simulink model "VB_RIFKF_GNSS_INS25"  (R2023a)
settings: Solver=FixedStepAuto  StartTime=0  StopTime=500  FixedStep=0.01  RelTol=1e-3
InitFcn:
  | resilient_initNavigation1216;
  | init_param;
undefined symbols (not defined in the file or in its folder): dt, g0, gam0_rad, ISUS_flag, magnitude, p, P0, P0_RIEKF, param, pd0, pe0, phi0_rad, pn0, psi, psi0_rad, state_dim, vd0, ve0, vn0
libraries: simulink_extras x68, dspstat3 x54, sharedtransform x47, simulink x43, matrix_library x9, sharedTrackingLibrary x5, dspfactors x4, aerolibconvert2 x3, aerolibtransform2 x3
(part 18 of 22)

== matlab function VB_RIFKF_GNSS_INS25/ER EKF/INS propogation/Init_PVQ/Horizontal_attitude2/Hem2JPL2 ==
  data: q input; y output
function y = fcn(q)

y = [q(2:4);q(1)];

== matlab function VB_RIFKF_GNSS_INS25/ER EKF/INS propogation/att_update/JPLQuatMult ==
  data: quatA input; q_t output; quatB input
function q_t = QuatMult(quatA,quatB)
% Calculate the following quaternion product quatA * quatB using the 
% standard identity 
%{
inline Eigen::Matrix<double, 4, 1> quat_multiply(const Eigen::Matrix<double, 4, 1> &q, const Eigen::Matrix<double, 4, 1> &p) {
  Eigen::Matrix<double, 4, 1> q_t;
  Eigen::Matrix<double, 4, 4> Qm;
  // create big L matrix
  Qm.block(0, 0, 3, 3) = q(3, 0) * Eigen::MatrixXd::Identity(3, 3) - skew_x(q.block(0, 0, 3, 1));
  Qm.block(0, 3, 3, 1) = q.block(0, 0, 3, 1);
  Qm.block(3, 0, 1, 3) = -q.block(0, 0, 3, 1).transpose();
  Qm(3, 3) = q(3, 0);
  q_t = Qm * p;
  // ensure unique by forcing q_4 to be >0
  if (q_t(3, 0) < 0) {
    q_t *= -1;
  }
  // normalize and return
  return q_t / q_t.norm();
}
%}
Qm = zeros(4,4);
q_t = zeros(4,1);
Qm(1:3,1:3) = quatA(4)*eye(3,3) - skewMat(quatA(1:3));
Qm(1:3,4) = quatA(1:3);
Qm(4,1:3) = -quatA(1:3)';
Qm(4,4) = quatA(4);
q_t = Qm * quatB;
if q_t(4) < 0
    q_t = q_t * (-1);
end
q_t = q_t / norm(q_t);
end

== matlab function VB_RIFKF_GNSS_INS25/ISUS_RIEKF3/INS propogation3/vel//pos update/pos update/MATLAB Function ==
  data: dtheta input; pos_correct output single; KFState_dp input; pos input
function pos_correct = fcn(dtheta, KFState_dp, pos)
    
     pos_correct =  KFState_dp + exp_so3(dtheta)*pos;
    %pos_correct = pos + KFState_dp - skewMat(pos)*dtheta;
    
end

== matlab function VB_RIFKF_GNSS_INS25/ER EKF/INS propogation/att_update/JPLQuatMult1 ==
  data: quatA input; q_t output; quatB input
function q_t = QuatMult(quatA,quatB)
% Calculate the following quaternion product quatA * quatB using the 
% standard identity 
%{
inline Eigen::Matrix<double, 4, 1> quat_multiply(const Eigen::Matrix<double, 4, 1> &q, const Eigen::Matrix<double, 4, 1> &p) {
  Eigen::Matrix<double, 4, 1> q_t;
  Eigen::Matrix<double, 4, 4> Qm;
  // create big L matrix
  Qm.block(0, 0, 3, 3) = q(3, 0) * Eigen::MatrixXd::Identity(3, 3) - skew_x(q.block(0, 0, 3, 1));
  Qm.block(0, 3, 3, 1) = q.block(0, 0, 3, 1);
  Qm.block(3, 0, 1, 3) = -q.block(0, 0, 3, 1).transpose();
  Qm(3, 3) = q(3, 0);
  q_t = Qm * p;
  // ensure unique by forcing q_4 to be >0
  if (q_t(3, 0) < 0) {
    q_t *= -1;
  }
  // normalize and return
  return q_t / q_t.norm();
}
%}
Qm = zeros(4,4);
q_t = zeros(4,1);
Qm(1:3,1:3) = quatA(4)*eye(3,3) - skewMat(quatA(1:3));
Qm(1:3,4) = quatA(1:3);
Qm(4,1:3) = -quatA(1:3)';
Qm(4,4) = quatA(4);
q_t = Qm * quatB;
if q_t(4) < 0
    q_t = q_t * (-1);
end
q_t = q_t / norm(q_t);
end

== matlab function VB_RIFKF_GNSS_INS25/ER EKF/INS propogation/att_update/JPLrv2q ==
  data: rotVec input; quaternion output
% convert froma rotation vector in radians to a quaternion
function quaternion = RotToQuat(rotVec)

vecLength = sqrt(rotVec(1)^2 + rotVec(2)^2 + rotVec(3)^2);

if vecLength < 1e-6
  quaternion = [0;0;0;1];
else
  quaternion = [rotVec/vecLength*sin(0.5*vecLength);cos(0.5*vecLength);];
end

== matlab function VB_RIFKF_GNSS_INS25/ER EKF/INS propogation/att_update/JPLrv2q1 ==
  data: deltaTheta input; updateQuat output
% convert froma rotation vector in radians to a quaternion
function updateQuat = RotToQuat(deltaTheta)

    deltaq = 0.5 * deltaTheta;
    
    checkNorm = deltaq' * deltaq;
    
    if checkNorm > 1
        updateQuat = [deltaq; 1];
        updateQuat = updateQuat / sqrt(1 + checkNorm);
    else
        updateQuat = [deltaq; sqrt(1 - checkNorm)];
    end
    
    updateQuat = updateQuat / norm(updateQuat);
end

== matlab function VB_RIFKF_GNSS_INS25/ER EKF/INS propogation/att_update/MATLAB Function1 ==
  data: q input; Rot output
function Rot = quat_2_Rot(q)

%{
inline Eigen::Matrix<double, 3, 3> quat_2_Rot(const Eigen::Matrix<double, 4, 1> &q) {
  Eigen::Matrix<double, 3, 3> q_x = skew_x(q.block(0, 0, 3, 1));
  Eigen::MatrixXd Rot = (2 * std::pow(q(3, 0), 2) - 1) * Eigen::MatrixXd::Identity(3, 3) - 2 * q(3, 0) * q_x +
                        2 * q.block(0, 0, 3, 1) * (q.block(0, 0, 3, 1).transpose());
  return Rot;
}
%}
q_x = skewMat(q(1:3));
Rot = (2 * q(4)^2 - 1) * eye(3, 3) - 2 * q(4) * q_x +...
       2 * q(1:3) * q(1:3)';
end

== matlab function VB_RIFKF_GNSS_INS25/ISUS_RIEKF3/Error State Kalman Filter M1/Extended Kalman Filter M1/Correct M1/Correct ==
  settings: updateMethod=DISCRETE  sampleTime=SampleTime
  data: x input; xNew output; P input; P output; yMeas input; R input; uMeas input; blockOrdering input; pM parameter; blockOrdering output
function [xNew,P,blockOrdering] = fcn(x,P,yMeas,R,uMeas,blockOrdering,pM)
% ekfCorrect Correction step for EKF
%
%   Copyright 2016-2021 The MathWorks, Inc.

%#codegen

% If measurement noise is time-varying then compute square-root
% factorization.
if pM.HasTimeVaryingR
   R = matlabshared.tracking.internal.svdPSD(R);
end

% Construct the function handle for measurement fcn
if pM.IsSimulinkFcn
    MeasurementFcnH_SL = str2func(pM.FcnName);
    if pM.HasAdditiveNoise
        MeasurementFcnH = @(fState)MeasurementFcnH_SL(fState);
    else
        MeasurementFcnH = @(fState,fMeasNoise)MeasurementFcnH_SL(fState,fMeasNoise);
    end
else
    MeasurementFcnH = str2func(pM.FcnName);
end

% Construct the function handle for measurement Jacobian fcn
if pM.HasJacobian
    if pM.IsSimulinkFcn
        MeasurementJacobianFcnH_SL = str2func(pM.JacobianFcnName);
        if pM.HasAdditiveNoise
            MeasurementJacobianFcnH = @(fState)MeasurementJacobianFcnH_SL(fState);
        else
            MeasurementJacobianFcnH = @(fState,fMeasNoise)MeasurementJacobianFcnH_SL(fState,fMeasNoise);
        end
    else
        MeasurementJacobianFcnH = str2func(pM.JacobianFcnName);
    end
else
    MeasurementJacobianFcnH = [];
end

% Handle (optional) extra input arguments of the measurement & jacobian fcns
switch pM.NumberOfExtraArgumentInports
    case 0
        extraArgs = {};
    case 1
        extraArgs = {uMeas};
    otherwise
        assert(false);
end

% Construct the corrector, perform the update
if pM.HasAdditiveNoise
    ekfCorrector = matlabshared.tracking.internal.EKFCorrectorAdditive();
else
    ekfCorrector = matlabshared.tracking.internal.EKFCorrectorNonAdditive();
end

% Check if dimensions and type of Measurement and Jacobian are correct
if pM.HasAdditiveNoise
   % Additive noise
   
   % MeasurementFcn
   ztry = MeasurementFcnH(x, extraArgs{:});
   
   if pM.IsSimulinkFcn
      hasError = (numel(ztry) ~= numel(yMeas));
   else
      hasError = (numel(ztry) ~= numel(yMeas)) || ~isa(ztry, class(x));
   end
   
   coder.internal.errorIf(...
      hasError,...
      'shared_tracking:ExtendedKalmanFilter:MeasurementNonMatchingSizeOrClass',...
      'MeasurementFcn');
   
   if pM.HasJacobian
      % MeasurementJacobianFcn
      Htry = MeasurementJacobianFcnH(x, extraArgs{:});
      isSizeNotCorrect = numel(yMeas) ~= size(Htry,1) || numel(x) ~= size(Htry,2);
      
      if pM.IsSimulinkFcn
         hasError = isSizeNotCorrect;
      else
         hasError = isSizeNotCorrect || ~isa(Htry, class(x));
      end
      
      coder.internal.errorIf(...
         hasError,...
         'shared_tracking:ExtendedKalmanFilter:MeasurementJacobianNonMatchingSizeOrClass',...
         'MeasurementJacobianFcn',numel(yMeas),numel(x));
   end   
else
   % Non-additive noise
   
   % MeasurementFcn
   ztry = MeasurementFcnH(...
      x, zeros(size(R,1),1,'like',x), ...
      extraArgs{:});   

   if pM.IsSimulinkFcn
      hasError = (numel(ztry) ~= numel(yMeas));
   else
      hasError = (numel(ztry) ~= numel(yMeas)) || ~isa(ztry, class(x));
   end
   
   coder.internal.errorIf(...
      hasError,...
      'shared_tracking:ExtendedKalmanFilter:MeasurementNonMatchingSizeOrClass',...
      'MeasurementFcn');
   
   if pM.HasJacobian
      % MeasurementJacobianFcn
      Htry = MeasurementJacobianFcnH(...
         x, zeros(size(R,1),1,'like',x), ...
         extraArgs{:});
      
      isSizeNotCorrect = numel(yMeas) ~= size(Htry,1) || numel(x) ~= size(Htry,2);     
      
      if pM.IsSimulinkFcn
         hasError = isSizeNotCorrect;
      else
         hasError = isSizeNotCorrect || ~isa(Htry, class(x));
      end
      
      coder.internal.errorIf(...
         hasError,...
         'shared_tracking:ExtendedKalmanFilter:MeasurementJacobianNonMatchingSizeOrClass',...
         'MeasurementJacobianFcn',numel(yMeas),numel(x));
   end
end
% Measurement wrapping
ekfCorrector.HasMeasurementWrapping = pM.HasWrapping;

xNew = zeros(size(x),'like',x); %#ok<PREALL>
% wk = 0;
[xNew,P] = ekfCorrector.correct(...
        yMeas,R,x,P,MeasurementFcnH,MeasurementJacobianFcnH,extraArgs{:});
end

== matlab function VB_RIFKF_GNSS_INS25/ISUS_RIEKF3/Error State Kalman Filter M1/Extended Kalman Filter M1/Correct M1/MATLAB Function ==
  data: u input; y output
function y = fcn(u)

y = tril(u);

== matlab function VB_RIFKF_GNSS_INS25/ISUS_RIEKF3/Error State Kalman Filter M1/Extended Kalman Filter M1/Correct M1/Subsystem2/MATLAB Function1 ==
  data: u input; y output; X input; ISUS_flag input
function y = fcn(u, X, ISUS_flag)
if ISUS_flag == 0
    y = X;
else
     y = u;
    %y(1:9,1:9) = u;
end

== matlab function VB_RIFKF_GNSS_INS25/ISUS_RIEKF3/Error State Kalman Filter M1/Extended Kalman Filter M1/Correct M1/innovation calculation/MATLAB Function ==
  data: u input; y output
function y = fcn(u)

y = u*u';

== matlab function VB_RIFKF_GNSS_INS25/ISUS_RIEKF3/Error State Kalman Filter M1/Extended Kalman Filter M1/Output/MATLAB Function ==
  data: S input; P output
function P = fcn(S)
    
    % Get back Covariance from Square-root Covariance
    P = S*S';
    %P = 1/2*(S+S');
    
end

== matlab function VB_RIFKF_GNSS_INS25/ISUS_RIEKF3/Error State Kalman Filter M1/Extended Kalman Filter M1/Predict/Predict ==
  settings: updateMethod=DISCRETE  sampleTime=SampleTime
  data: x input; xNew output; P input; Q input; uState input; unused input; P output; pS parameter
function [xNew,P] = fcn(x,P,Q,uState,~,pS)
% ekfCorrect Prediction step for EKF
%
%   Copyright 2016-2021 The MathWorks, Inc.

%#codegen

% If process noise is time-varying then compute square-root
% factorization.
if pS.HasTimeVaryingQ
   Q = matlabshared.tracking.internal.svdPSD(Q);
end

% Construct fcn handles
if pS.IsSimulinkFcn
    StateTransitionJacobianFcnH_SL = str2func(pS.FcnName);
    if pS.HasAdditiveNoise
        StateTransitionFcnH = @(fState)StateTransitionJacobianFcnH_SL(fState);
    else
        StateTransitionFcnH = @(fState,fProcNoise)StateTransitionJacobianFcnH_SL(fState,fProcNoise);
    end
else
    StateTransitionFcnH = str2func(pS.FcnName);
end
if pS.HasJacobian
    if pS.IsSimulinkFcn
        StateTransitionJacobianFcnH_SL = str2func(pS.JacobianFcnName);
        if pS.HasAdditiveNoise
            StateTransitionJacobianFcnH = @(fState)StateTransitionJacobianFcnH_SL(fState);
        else
            StateTransitionJacobianFcnH = @(fState,fProcNoise)StateTransitionJacobianFcnH_SL(fState,fProcNoise);
        end
    else
        StateTransitionJacobianFcnH = str2func(pS.JacobianFcnName);
    end
else
    StateTransitionJacobianFcnH = [];
end

switch pS.NumberOfExtraArgumentInports
    case 0
        extraArgs = {};
    case 1
        extraArgs = {uState};
    otherwise
        assert(false);
end

% Check if dimensions and type of State and Jacobian are correct
if pS.HasAdditiveNoise
   % Additive noise
   
   % StateTransitionFcn
   xTry = StateTransitionFcnH(x, extraArgs{:});
   
   if pS.IsSimulinkFcn
      hasError = any(size(x) ~= size(xTry));
   else
      hasError = any(size(x) ~= size(xTry)) || ~isa(xTry, class(x));
   end
   
   coder.internal.errorIf(...
      hasError,...
      'shared_tracking:ExtendedKalmanFilter:StateNonMatchingSizeOrClass',...
      'StateTransitionFcn', 'State', numel(x));
   
   if pS.HasJacobian
      % Jacobian
      F = StateTransitionJacobianFcnH(x, extraArgs{:});
      % F needs to be square
      isSizeNotCorrect = ~all(size(F) == numel(x));
      
      if pS.IsSimulinkFcn
         hasError = isSizeNotCorrect;
      else
         hasError = isSizeNotCorrect || ~isa(F, class(x));
      end
      
      coder.internal.errorIf(...
         hasError,...
         'shared_tracking:ExtendedKalmanFilter:StateTransitionJacobianNonMatchingSizeOrClass',...
         'StateTransitionJacobianFcn', numel(x));
   end
else
   % Non-additive noise
   
   % StateTransitionFcn
   xTry = StateTransitionFcnH(x, zeros(size(Q,1),1,'like',x),extraArgs{:});
   
   if pS.IsSimulinkFcn
      hasError = any(size(x) ~= size(xTry));
   else
      hasError = any(size(x) ~= size(xTry)) || ~isa(xTry, class(x));
   end
   
   coder.internal.errorIf(...
      hasError,...
      'shared_tracking:ExtendedKalmanFilter:StateNonMatchingSizeOrClass',...
      'StateTransitionFcn', 'State', numel(x))
   
   if pS.HasJacobian
      % Jacobian
      F = StateTransitionJacobianFcnH(x, zeros(size(Q,1),1,'like',x),extraArgs{:});
      % F needs to be square
      isSizeNotCorrect = ~all(size(F) == numel(x));
      
      if pS.IsSimulinkFcn
         hasError = isSizeNotCorrect;
      else
         hasError = isSizeNotCorrect || ~isa(F, class(x));
      end
       
      coder.internal.errorIf(...
         hasError,...
         'shared_tracking:ExtendedKalmanFilter:StateTransitionJacobianNonMatchingSizeOrClass',...
         'StateTransitionJacobianFcn', numel(x));
   end
end

xNew = zeros(size(x),'like',x); %#ok<PREALL>

if pS.HasAdditiveNoise
    [xNew,P] = matlabshared.tracking.internal.EKFPredictorAdditive.predict(...
        Q,x,P,StateTransitionFcnH,StateTransitionJacobianFcnH,extraArgs{:});
else    
    [xNew,P] = matlabshared.tracking.internal.EKFPredictorNonAdditive.predict(...
        Q,x,P,StateTransitionFcnH,StateTransitionJacobianFcnH,extraArgs{:});
end
end

== matlab function VB_RIFKF_GNSS_INS25/ISUS_RIEKF3/Error State Kalman Filter M1/Extended Kalman Filter M1/innovation calculation/MATLAB Function ==
  data: u input; y output
function y = fcn(u)

y = u*u';

== matlab function VB_RIFKF_GNSS_INS25/ER EKF/Error State Kalman Filter/Extended Kalman Filter2/Correct1/Correct ==
  settings: updateMethod=DISCRETE  sampleTime=SampleTime
  data: x input; xNew output; P input; P output; yMeas input; R input; uMeas input; blockOrdering input; pM parameter; blockOrdering output
function [xNew,P,blockOrdering] = fcn(x,P,yMeas,R,uMeas,blockOrdering,pM)
% ekfCorrect Correction step for EKF
%
%   Copyright 2016-2021 The MathWorks, Inc.

%#codegen

% If measurement noise is time-varying then compute square-root
% factorization.
if pM.HasTimeVaryingR
   R = matlabshared.tracking.internal.svdPSD(R);
end

% Construct the function handle for measurement fcn
if pM.IsSimulinkFcn
    MeasurementFcnH_SL = str2func(pM.FcnName);
    if pM.HasAdditiveNoise
        MeasurementFcnH = @(fState)MeasurementFcnH_SL(fState);
    else
        MeasurementFcnH = @(fState,fMeasNoise)MeasurementFcnH_SL(fState,fMeasNoise);
    end
else
    MeasurementFcnH = str2func(pM.FcnName);
end

% Construct the function handle for measurement Jacobian fcn
if pM.HasJacobian
    if pM.IsSimulinkFcn
        MeasurementJacobianFcnH_SL = str2func(pM.JacobianFcnName);
        if pM.HasAdditiveNoise
            MeasurementJacobianFcnH = @(fState)MeasurementJacobianFcnH_SL(fState);
        else
            MeasurementJacobianFcnH = @(fState,fMeasNoise)MeasurementJacobianFcnH_SL(fState,fMeasNoise);
        end
    else
        MeasurementJacobianFcnH = str2func(pM.JacobianFcnName);
    end
else
    MeasurementJacobianFcnH = [];
end

% Handle (optional) extra input arguments of the measurement & jacobian fcns
switch pM.NumberOfExtraArgumentInports
    case 0
        extraArgs = {};
    case 1
        extraArgs = {uMeas};
    otherwise
        assert(false);
end

% Construct the corrector, perform the update
if pM.HasAdditiveNoise
    ekfCorrector = matlabshared.tracking.internal.EKFCorrectorAdditive();
else
    ekfCorrector = matlabshared.tracking.internal.EKFCorrectorNonAdditive();
end

% Check if dimensions and type of Measurement and Jacobian are correct
if pM.HasAdditiveNoise
   % Additive noise
   
   % MeasurementFcn
   ztry = MeasurementFcnH(x, extraArgs{:});
   
   if pM.IsSimulinkFcn
      hasError = (numel(ztry) ~= numel(yMeas));
   else
      hasError = (numel(ztry) ~= numel(yMeas)) || ~isa(ztry, class(x));
   end
   
   coder.internal.errorIf(...
      hasError,...
      'shared_tracking:ExtendedKalmanFilter:MeasurementNonMatchingSizeOrClass',...
      'MeasurementFcn');
   
   if pM.HasJacobian
      % MeasurementJacobianFcn
      Htry = MeasurementJacobianFcnH(x, extraArgs{:});
      isSizeNotCorrect = numel(yMeas) ~= size(Htry,1) || numel(x) ~= size(Htry,2);
      
      if pM.IsSimulinkFcn
         hasError = isSizeNotCorrect;
      else
         hasError = isSizeNotCorrect || ~isa(Htry, class(x));
      end
      
      coder.internal.errorIf(...
         hasError,...
         'shared_tracking:ExtendedKalmanFilter:MeasurementJacobianNonMatchingSizeOrClass',...
         'MeasurementJacobianFcn',numel(yMeas),numel(x));
   end   
else
   % Non-additive noise
   
   % MeasurementFcn
   ztry = MeasurementFcnH(...
      x, zeros(size(R,1),1,'like',x), ...
      extraArgs{:});   

   if pM.IsSimulinkFcn
      hasError = (numel(ztry) ~= numel(yMeas));
   else
      hasError = (numel(ztry) ~= numel(yMeas)) || ~isa(ztry, class(x));
   end
   
   coder.internal.errorIf(...
      hasError,...
      'shared_tracking:ExtendedKalmanFilter:MeasurementNonMatchingSizeOrClass',...
      'MeasurementFcn');
   
   if pM.HasJacobian
      % MeasurementJacobianFcn
      Htry = MeasurementJacobianFcnH(...
         x, zeros(size(R,1),1,'like',x), ...
         extraArgs{:});
      
      isSizeNotCorrect = numel(yMeas) ~= size(Htry,1) || numel(x) ~= size(Htry,2);     
      
      if pM.IsSimulinkFcn
         hasError = isSizeNotCorrect;
      else
         hasError = isSizeNotCorrect || ~isa(Htry, class(x));
      end
      
      coder.internal.errorIf(...
         hasError,...
         'shared_tracking:ExtendedKalmanFilter:MeasurementJacobianNonMatchingSizeOrClass',...
         'MeasurementJacobianFcn',numel(yMeas),numel(x));
   end
end
% Measurement wrapping
ekfCorrector.HasMeasurementWrapping = pM.HasWrapping;

xNew = zeros(size(x),'like',x); %#ok<PREALL>
% wk = 0;
[xNew,P] = ekfCorrector.correct(...
        yMeas,R,x,P,MeasurementFcnH,MeasurementJacobianFcnH,extraArgs{:});
end

== matlab function VB_RIFKF_GNSS_INS25/ISUS_RIEKF3/Error State Kalman Filter M1/MATLAB Function ==
  data: u input; dp output size=3; dv output size=3; dtheta output size=3; da output size=3; dg output size=3
function [dp,dv,dtheta,da,dg] = fcn(u)
    dtheta = u(1:3);
    dv = u(4:6);
    dp = u(7:9);
    dg = u(10:12);
    da = u(13:15);

end

== matlab function VB_RIFKF_GNSS_INS25/ISUS_RIEKF1/INS propogation/att update/MATLAB Function ==
  data: Rbn_k_1 input; Rbn output; w input; dt input
function Rbn = fcn(Rbn_k_1, w, dt)
    Rbn =  Rbn_k_1 * exp_so3( w * dt);
end

== matlab function VB_RIFKF_GNSS_INS25/ISUS_RIEKF1/INS propogation/att update/MATLAB Function2 ==
  data: delta input; Rbn_correct output single size=[3,3]; Rbn input
function Rbn_correct = fcn(delta, Rbn)
    Rbn_correct = zeros(3,3);
     Rbn_correct = exp_so3(delta)* Rbn;
    %Rbn_correct =( eye(3) + skewMat(delta))* Rbn;
end

== matlab function VB_RIFKF_GNSS_INS25/ISUS_RIEKF1/INS propogation/vel//pos update/pos update/MATLAB Function ==
  data: dtheta input; pos_correct output single; KFState_dp input; pos input
function pos_correct = fcn(dtheta, KFState_dp, pos)
    
     pos_correct =  KFState_dp + exp_so3(dtheta)*pos;
    %pos_correct = pos + KFState_dp - skewMat(pos)*dtheta;
    
end

== matlab function VB_RIFKF_GNSS_INS25/ISUS_RIEKF1/INS propogation/vel//pos update/vel update/MATLAB Function ==
  data: dtheta input; vel_correct output single; KFState_dv input; vel input
function vel_correct = fcn(dtheta, KFState_dv, vel)
    
     vel_correct =  KFState_dv + exp_so3( dtheta)*vel;
    %vel_correct =  vel + KFState_dv - skewMat(vel)*dtheta;
end

== matlab function VB_RIFKF_GNSS_INS25/ISUS_RIEKF3/Error State Kalman Filter M1/Simulink Function - GPS Measurements/MATLAB Function ==
  data: vn input; H output; pn input
function H = fcn(vn, pn)
    state_dim = 15;
    H = zeros(6,state_dim);
    H(1:3,1:3) = skewMat(vn);
    H(4:6,1:3) = skewMat(pn);
    H(1:6,4:9) = eye(6);
    %H = -H;
end

== matlab function VB_RIFKF_GNSS_INS25/ISUS_RIEKF3/Error State Kalman Filter M1/Simulink Function - GPS Measurements/MATLAB Function1 ==
  data: Rbn input; vn input; X_inv output; pn input
function X_inv = invX(Rbn, vn, pn)
    X_inv = zeros(5,5);
    Rnb = Rbn';
    X_inv(1:3,1:3) = Rnb;
    X_inv(1:3,4) = -Rnb * vn;
    X_inv(1:3,5) = -Rnb * pn;
    X_inv(4:5,4:5) = eye(2);
end

== matlab function VB_RIFKF_GNSS_INS25/ISUS_RIEKF3/Error State Kalman Filter M1/Simulink Function - GPS Measurements1/MATLAB Function ==
  data: vn input; H_baro output; pn input
function H_baro = fcn(vn, pn)
    state_dim = 24;
    H = zeros(6,state_dim);
    H(1:3,1:3) = skewMat(vn);
    H(4:6,1:3) = skewMat(pn);
    H(1:6,4:9) = eye(6);
    
    A = [0 0 0 0 0 1];
    H_baro = A * H;
end

== matlab function VB_RIFKF_GNSS_INS25/ISUS_RIEKF3/Error State Kalman Filter M1/Simulink Function - GPS Measurements2/MATLAB Function ==
  data: Rbn input; Magn input; H output; dtheta input
function H = fcn(Rbn, Magn, dtheta)
    state_dim = 24;
    H = zeros(3,state_dim);
    H(1:3,1:3) =  Rbn * skewMat(Magn);
    H(1:3,16:18) =  Rbn * skewMat(dtheta);
end

== matlab function VB_RIFKF_GNSS_INS25/ISUS_RIEKF3/Error State Kalman Filter M1/Simulink Function - GPS Measurements3/MATLAB Function ==
  data: Rbn input; Rab input; H output; vn input; v_wind input
function H = fcn(Rbn,Rab, vn,v_wind)
    state_dim = 24;
    A = Rab' * Rbn';
    H = zeros(3,state_dim);
   % H(1:3,1:3) =  - skewMat(vn - v_wind);
   % H(1:3,4:6) =  eye(3);
    H(1:3,19:21) =  - skewMat(vn - v_wind);
    H(1:3,22:24) =  - eye(3);
    H = double(A * H);
end

== matlab function VB_RIFKF_GNSS_INS25/ISUS_RIEKF3/Error State Kalman Filter M1/Simulink Function - State Transition/Cal Phi/MATLAB Function1 ==
  data: vn input; Phi output; pn input; Rbn input; dt input
function Phi = fcn(vn,pn, Rbn,dt)
    state_dim = 15;
    %{
    F.block(0, 0, 3, 3) = exp_so3(-w_hat * dt);
        F.block(0, 9, 3, 3).noalias() = -exp_so3(-w_hat * dt) * Jr_so3(-w_hat * dt) * dt;
        F.block(9, 9, 3, 3).setIdentity();
        F.block(6, 0, 3, 3).noalias() = -R_Gtoi.transpose() * skew_x(a_hat * dt);
        F.block(6, 6, 3, 3).setIdentity();
        F.block(6, 12, 3, 3) = -R_Gtoi.transpose() * dt;
        F.block(12, 12, 3, 3).setIdentity();
        F.block(3, 0, 3, 3).noalias() = -0.5 * R_Gtoi.transpose() * skew_x(a_hat * dt * dt);
        F.block(3, 6, 3, 3) = Eigen::Matrix3d::Identity() * dt;
        F.block(3, 12, 3, 3) = -0.5 * R_Gtoi.transpose() * dt * dt;
        F.block(3, 3, 3, 3).setIdentity();
        Eigen::Matrix<double, 15, 12> G = Eigen::Matrix<double, 15, 12>::Zero();
    %}
    %
    %
    %F = [0_33         0_33  0_33   -Rbn          0_33]
    %    [skew(gn)     0_33  0_33  -skew(vn)Rbn   -Rbn]
    %    [0.5*skew(gn) I_33  0_33  -skew(pn)Rbn   -Rbn]
    %    [         0_69                  I66          ]
    %
    %0611 yxy
        %F = [0_33         0_33  0_33   -Rbn          0_33]
    %    [skew(gn)     0_33  0_33  -skew(vn)Rbn   Rbn]
    %    [0.5*skew(gn) I_33  0_33  -skew(pn)Rbn   Rbn]
    %    [         0_69                  I66          ]
    Phi = zeros(state_dim,state_dim);
    g0 = 9.79;
    gn = [0;0;-g0];
    tao_wind = 50;
    F  = zeros(state_dim,state_dim);
    F(1:3,10:12) = -Rbn;
    F(4:6,1:3)   = skewMat(gn);
    F(4:6,10:12) = -skewMat(vn)*Rbn;
    F(4:6,13:15) = -Rbn*(-1);
    F(7:9,4:6)   = eye(3);
    F(7:9,1:3)   = 0.5*skewMat(gn)*dt;
    F(7:9,10:12) = -skewMat(pn)*Rbn;
    F(7:9,13:15) = -Rbn*(-1);
    %F(10:15,10:15) = eye(6);
    % F(22:24,22:24) = -1/tao_wind;
    Phi = eye(state_dim) + F * dt;

end

== matlab function VB_RIFKF_GNSS_INS25/ISUS_RIEKF3/Error State Kalman Filter M1/Simulink Function - State Transition/MATLAB Function ==
  data: Rbn input; G output; vn input; pn input; dt input
function G = fcn(Rbn, vn,pn, dt)
    % G.block(0, 0, 3, 3) = -exp_so3(-w_hat * dt) * Jr_so3(-w_hat * dt) * dt;
    %    G.block(6, 3, 3, 3) = -R_Gtoi.transpose() * dt;
    %    G.block(3, 3, 3, 3) = -0.5 * R_Gtoi.transpose() * dt * dt;
    %    G.block(9, 6, 3, 3).setIdentity();
    %    G.block(12, 9, 3, 3).setIdentity();
    state_dim = 15;
    cov_dim = 12;
    G = zeros(state_dim,cov_dim);
    % G(1:3,1:3) = -  Rbn * dt;
    % G(4:6,1:3) = -skewMat(vn)*Rbn* dt;
    % G(4:6,4:6) =  - Rbn;
    % G(7:9,1:3) = -skewMat(pn)*Rbn * dt;
    % G(7:9,4:6) =  - Rbn;
    % G(10:12,7:9) = eye(3)*dt;
    % G(13:15,10:12) = eye(3)*dt;
    G(1:3,1:3) =  - Rbn * dt;
    G(4:6,1:3) = -skewMat(vn)*Rbn * dt*(-1);
    G(4:6,4:6) =  - Rbn * dt;
    G(7:9,1:3) = -skewMat(pn)*Rbn * dt*(-1);
    G(7:9,4:6) =  - Rbn * dt;
    G(10:12,7:9) = eye(3)* dt;
    G(13:15,10:12) = eye(3);
    % G(16:18,13:15) = eye(3);
    % G(19:21,16:18) = eye(3)* dt;
    % G(22:24,19:21) = eye(3)* dt;
    %G = G*double(dt);
end

== matlab function VB_RIFKF_GNSS_INS25/ISUS_RIEKF3/Error State Kalman Filter M1/Simulink Function - State Transition1/Cal Phi/MATLAB Function1 ==
  data: vn input; Phi output; pn input; Rbn input; dt input
function Phi = fcn(vn,pn, Rbn,dt)
    state_dim = 15;
    %{
    F.block(0, 0, 3, 3) = exp_so3(-w_hat * dt);
        F.block(0, 9, 3, 3).noalias() = -exp_so3(-w_hat * dt) * Jr_so3(-w_hat * dt) * dt;
        F.block(9, 9, 3, 3).setIdentity();
        F.block(6, 0, 3, 3).noalias() = -R_Gtoi.transpose() * skew_x(a_hat * dt);
        F.block(6, 6, 3, 3).setIdentity();
        F.block(6, 12, 3, 3) = -R_Gtoi.transpose() * dt;
        F.block(12, 12, 3, 3).setIdentity();
        F.block(3, 0, 3, 3).noalias() = -0.5 * R_Gtoi.transpose() * skew_x(a_hat * dt * dt);
        F.block(3, 6, 3, 3) = Eigen::Matrix3d::Identity() * dt;
        F.block(3, 12, 3, 3) = -0.5 * R_Gtoi.transpose() * dt * dt;
        F.block(3, 3, 3, 3).setIdentity();
        Eigen::Matrix<double, 15, 12> G = Eigen::Matrix<double, 15, 12>::Zero();
    %}
    %
    %
    %F = [0_33         0_33  0_33   -Rbn          0_33]
    %    [skew(gn)     0_33  0_33  -skew(vn)Rbn   -Rbn]
    %    [0.5*skew(gn) I_33  0_33  -skew(pn)Rbn   -Rbn]
    %    [         0_69                  I66          ]
    %
    %0611 yxy
        %F = [0_33         0_33  0_33   -Rbn          0_33]
    %    [skew(gn)     0_33  0_33  -skew(vn)Rbn   Rbn]
    %    [0.5*skew(gn) I_33  0_33  -skew(pn)Rbn   Rbn]
    %    [         0_69                  I66          ]
    Phi = zeros(state_dim,state_dim);
    g0 = 9.79;
    gn = [0;0;-g0];
    tao_wind = 50;
    F  = zeros(state_dim,state_dim);
    F(1:3,10:12) = -Rbn;
    F(4:6,1:3)   = skewMat(gn);
    F(4:6,10:12) = -skewMat(vn)*Rbn;
    F(4:6,13:15) = -Rbn*(-1);
    F(7:9,4:6)   = eye(3);
    F(7:9,1:3)   = 0.5*skewMat(gn)*dt;
    F(7:9,10:12) = -skewMat(pn)*Rbn;
    F(7:9,13:15) = -Rbn*(-1);
    %F(10:15,10:15) = eye(6);
    % F(22:24,22:24) = -1/tao_wind;
    Phi = double(eye(state_dim) + F * dt);

end

== matlab function VB_RIFKF_GNSS_INS25/ISUS_RIEKF3/Error State Kalman Filter M1/Simulink Function - State Transition1/MATLAB Function ==
  data: Rbn input; G output; vn input; pn input; dt input
function G = fcn(Rbn, vn,pn, dt)
    % G.block(0, 0, 3, 3) = -exp_so3(-w_hat * dt) * Jr_so3(-w_hat * dt) * dt;
    %    G.block(6, 3, 3, 3) = -R_Gtoi.transpose() * dt;
    %    G.block(3, 3, 3, 3) = -0.5 * R_Gtoi.transpose() * dt * dt;
    %    G.block(9, 6, 3, 3).setIdentity();
    %    G.block(12, 9, 3, 3).setIdentity();
    state_dim = 15;
    cov_dim = 12;
    G = zeros(state_dim,cov_dim);
    % G(1:3,1:3) = -  Rbn * dt;
    % G(4:6,1:3) = -skewMat(vn)*Rbn* dt;
    % G(4:6,4:6) =  - Rbn;
    % G(7:9,1:3) = -skewMat(pn)*Rbn * dt;
    % G(7:9,4:6) =  - Rbn;
    % G(10:12,7:9) = eye(3)*dt;
    % G(13:15,10:12) = eye(3)*dt;
    G(1:3,1:3) =  - Rbn * dt;
    G(4:6,1:3) = -skewMat(vn)*Rbn * dt*(-1);
    G(4:6,4:6) =  - Rbn * dt;
    G(7:9,1:3) = -skewMat(pn)*Rbn * dt*(-1);
    G(7:9,4:6) =  - Rbn * dt;
    G(10:12,7:9) = eye(3)* dt;
    G(13:15,10:12) = eye(3);
    % G(16:18,13:15) = eye(3);
    % G(19:21,16:18) = eye(3)* dt;
    % G(22:24,19:21) = eye(3)* dt;
    %G = G*double(dt);
end

== matlab function VB_RIFKF_GNSS_INS25/ISUS_RIEKF3/Error State Kalman Filter M1/bak/MATLAB Function1 ==
  data: Cbn input; wxyz input; ZeroVelDetectFlag output; fbxyz input; fex input; ZeroVelDetectFlagold output
function [ZeroVelDetectFlag,ZeroVelDetectFlagold]  = ZeroVelDetect(Cbn, wxyz,fbxyz, fex)
%% Use buffer to restore IMU data
    Windows = 8;
    tao = 0.8;
    ZeroVelDetectFlag = false;
    ZeroVelDetectFlagold = false;
    persistent w_;
    persistent a_;
    
    if isempty(w_) && isempty(a_)
        w_ = single(zeros(3,Windows));
        a_ = single(zeros(3,Windows));
    end
    w_ = [w_(:,2:Windows),wxyz];
    a_ = [a_(:,2:Windows),fbxyz];
    
    g=9.79;

    sigma2_a = 0.009^2;
    sigma2_g = 0.025^2;
    %sigma2_fex = 0.01^2;
    T = single(0);
    T_old = single(0);
    
    ya_m=mean(a_,2);
    for k=Windows-1
         tmp_old=a_(:,k)-g*ya_m/norm(ya_m);
        
        T_old = T_old + w_(:,k)'*w_(:,k)/sigma2_g+tmp_old'*tmp_old/sigma2_a;
        T = T + w_(:,k)'*w_(:,k)/sigma2_g;
        T_old = T_old + w_(:,k)'*w_(:,k)/sigma2_g;
    end
    T=T/Windows;
    T_old=T_old/Windows;
    T_fex = (fex + Cbn'*[0;0;g])'*(fex + Cbn'*[0;0;g]);
    T = T + T_fex;
    w = w_;
    a = a_;

    if T < tao 
        ZeroVelDetectFlag = true;
    end
    if T_old < tao 
        ZeroVelDetectFlagold = true;
    end
end

== matlab function VB_RIFKF_GNSS_INS25/ISUS_RIEKF3/Error State Kalman Filter M1/bak/RIEKF ==
  data: Rbn input; vn input; pn input; bg input; ba input; phi input; Q input; P input; dt input; GNSS_Mea input; GNSS_flag input; Rbn_update output; vn_update output; pn_update output; bg_update output; ba_update output; cov output
function [Rbn_update,vn_update,pn_update,bg_update,ba_update,cov] = RIEKF(Rbn,vn,pn,bg,ba,phi,Q,P,dt,GNSS_Mea,GNSS_flag)
    %initial state
    state.Rbn = Rbn;
    state.vn = vn;
    state.pn = pn;
    state.bg = bg;
    state.ba = ba;
    state = Construct_State(state);
    %initial RIEKF filter 
    RIEKF.P = P;
    RIEKF.phi = phi;
%% Error State Predict
    RIEKF.Qk = RIEKF.phi * Q * RIEKF.phi' * dt;             %Qk = φ·Q·φ·δt
    RIEKF.P = RIEKF.phi * RIEKF.P * RIEKF.phi' + RIEKF.Qk;  %P = φ·P·φ + Qk
    RIEKF.H_GNSS = calH(state.vn, state.pn);                %H
    RIEKF.Y = GNSS_Mea;
    RIEKF.b_GNSS = [zeros(1,2);eye(2)]; %    [0 0]
                                        %b = [1 0]
                                        %    [0 1]
    RIEKF.noise_GNSS = diag([0.01*ones(3,1);0.01*ones(3,1)]); %set GNSS error conv
%%
    if (GNSS_flag == 1)
        [state,RIEKF] = GNSSupdate(state,RIEKF);
    end
    Rbn_update = state.Rbn;
    vn_update = state.vn;
    pn_update = state.pn;
    bg_update = state.bg;
    ba_update = state.ba;
    cov = RIEKF.P;
end

function state = Construct_State(state)
            state.X = zeros(5,5);
            state.X(1:5,1:5) = [state.Rbn, state.vn, state.pn; 
                            zeros(1,3),1,0; 
                            zeros(1,3),0,1;];
            % Add Landmarks
            % Parameters
           state.bias = [state.bg; state.ba];
end

function [state,RIEKF] = GNSSupdate(state,RIEKF)
    % correct
    S = RIEKF.H_GNSS  * RIEKF.P * RIEKF.H_GNSS' + RIEKF.noise_GNSS; %噪声R矩阵的处理是否需要变换？
    K = (RIEKF.P * RIEKF.H_GNSS')/S;
    innonation = state.X * RIEKF.Y - RIEKF.b_GNSS;

    delta = K * innonation;
    dX = expMat(delta(1:end-6));
    dbias = delta(end-5:end);
    state.X = dX * state.X;
    state.bias = state.bias + dbias;
    state = updatestate(state);
    I = eye(size(RIEKF.P));
    RIEKF.P = (I - K*RIEKF.H_GNSS )* RIEKF.P *(I - K*RIEKF.H_GNSS )' + K*RIEKF.noise_GNSS*K';
end

function eX = expMat(delta)
    eX = zeros(5,5);
    eX(1:3,1:3) = exp_so3(delta(1:3));
    eX(1:3,4) = reshape(delta(4:6),3,1);
    eX(1:3,5) = reshape(delta(7:9),3,1);
    eX(4,4) = 1;
    eX(5,5) = 1;
end

function R = exp_so3(w)
    w_x  = [0, -w(3), w(2);
            w(3), 0, -w(1);
            -w(2), w(1), 0];
    theta = norm(w);
    if theta < 1e-7
        A = 1;
        B = 0.5;
    else
        A = double(sin(theta) / theta);
        B = double((1 - cos(theta)) / (theta * theta));
    end
    
    if theta == 0
        R = double(eye(3));
    else
        R = double(eye(3) + A * w_x + B * w_x * w_x);
    end
end

function H = calH(vn, pn)
    H = zeros(6,15);
    H(1:3,1:3) = -skewMat(vn);
    H(4:6,1:3) = -skewMat(pn);
    H(1:6,4:9) = eye(6);
end

function state = updatestate(state)
        state.Rbn = state.X(1:3,1:3);
        state.vn = state.X(1:3,4);
        state.pn = state.X(1:3,5);
        state.bg = state.bias(1:3);
        state.ba = state.bias(4:6);
end

== matlab function VB_RIFKF_GNSS_INS25/No.1_Sensor_Data_Process/IMU_Data_Process/accl_preprocessing2/MATLAB Function2 ==
  data: curr_input input; curr_output output single; sample_freq input; cutoff_freq input
function curr_output = second_LPF_Butter_x(curr_input,sample_freq,cutoff_freq)
   persistent input_x;
   persistent output_x;

   if isempty(input_x)
       input_x = [0;0;0];
   end
   
   if isempty(output_x)
       output_x = [0;0;0];
   end
    B = [0,0,0];
    A = [0,0,0];
    M_PI_F = 3.1415926;
	fr = sample_freq / cutoff_freq;
	ohm = tan( M_PI_F / fr );
	c = 1.0 + 2.0 * cos( M_PI_F / 4.0 ) * ohm + ohm * ohm;
	B(1) = ohm * ohm / c;
	B(2) = 2.0 * B(1);
	B(3) = B(1);
	A(1) = 2.0 * ( ohm * ohm - 1.0) / c;
	A(2) = (1.0 - 2.0 * cos( M_PI_F / 4.0 ) * ohm + ohm * ohm) / c;
	%/*获取最新输入*/
	input_x(3) = curr_input;
	%/* Butterworth */
	output_x(3) =B(1) * input_x(3) + B(2) * input_x(2) +B(3) * input_x(1) - A(1) * output_x(2) - A(2) * output_x(1);
	curr_output = single(output_x(3));
   % /* 输入序列保存 */
	input_x(1) = input_x(2);
	input_x(2) = input_x(3);
	%/*输出序列保存 */
	output_x(1) = output_x(2);
	output_x(2) = output_x(3);

== matlab function VB_RIFKF_GNSS_INS25/ISUS_RIEKF3/Error State Kalman Filter M1/bak/Simulink Function - GPS Measurements1/MATLAB Function1 ==
  data: H output; Cbn input; dt input
function H = calH(Cbn, dt)
    

    H = zeros(3,18);
    % 

    H(1:3,4:6) = eye(3);
    H(1:3,16:18) = -Cbn * dt;
end

== matlab function VB_RIFKF_GNSS_INS25/ISUS_RIEKF3/Error State Kalman Filter M1/bak/Simulink Function - State Transition Jacobian/Cal Phi1/MATLAB Function1 ==
  data: vn input; Phi output; pn input; Rbn input; dt input
function Phi = fcn(vn,pn, Rbn,dt)
    
    %{
    F.block(0, 0, 3, 3) = exp_so3(-w_hat * dt);
        F.block(0, 9, 3, 3).noalias() = -exp_so3(-w_hat * dt) * Jr_so3(-w_hat * dt) * dt;
        F.block(9, 9, 3, 3).setIdentity();
        F.block(6, 0, 3, 3).noalias() = -R_Gtoi.transpose() * skew_x(a_hat * dt);
        F.block(6, 6, 3, 3).setIdentity();
        F.block(6, 12, 3, 3) = -R_Gtoi.transpose() * dt;
        F.block(12, 12, 3, 3).setIdentity();
        F.block(3, 0, 3, 3).noalias() = -0.5 * R_Gtoi.transpose() * skew_x(a_hat * dt * dt);
        F.block(3, 6, 3, 3) = Eigen::Matrix3d::Identity() * dt;
        F.block(3, 12, 3, 3) = -0.5 * R_Gtoi.transpose() * dt * dt;
        F.block(3, 3, 3, 3).setIdentity();
        Eigen::Matrix<double, 15, 12> G = Eigen::Matrix<double, 15, 12>::Zero();
    %}
    %
    %
    %F = [0_33         0_33  0_33   -Rbn          0_33]
    %    [skew(gn)     0_33  0_33  -skew(vn)Rbn   -Rbn]
    %    [0.5*skew(gn) I_33  0_33  -skew(pn)Rbn   -Rbn]
    %    [         0_69                  I66          ]
    Phi = zeros(15,15);
    g0 = 9.79;
    gn = [0;0;-g0];
    F  = zeros(15,15);
    F(1:3,10:12) = -Rbn;
    F(4:6,1:3)   = skewMat(gn);
    F(4:6,10:12) = -skewMat(vn)*Rbn;
    F(4:6,13:15) = -Rbn;
    F(7:9,4:6)   = eye(3);
    F(7:9,1:3)   = 0.5*skewMat(gn) * dt;
    F(7:9,10:12) = -skewMat(pn)*Rbn;
    F(7:9,13:15) = -Rbn;
    %F(10:15,10:15) = eye(6);
    Phi = eye(15) + F * dt;

end

== matlab function VB_RIFKF_GNSS_INS25/ISUS_RIEKF3/Error State Kalman Filter M1/bak/Simulink Function - State Transition Jacobian/MATLAB Function1 ==
  data: Rbn input; G output; vn input; pn input; dt input
function G = fcn(Rbn, vn,pn, dt)
    % G.block(0, 0, 3, 3) = -exp_so3(-w_hat * dt) * Jr_so3(-w_hat * dt) * dt;
    %    G.block(6, 3, 3, 3) = -R_Gtoi.transpose() * dt;
    %    G.block(3, 3, 3, 3) = -0.5 * R_Gtoi.transpose() * dt * dt;
    %    G.block(9, 6, 3, 3).setIdentity();
    %    G.block(12, 9, 3, 3).setIdentity();

    G = zeros(15,12);
    % G(1:3,1:3) = -  Rbn * dt;
    % G(4:6,1:3) = -skewMat(vn)*Rbn* dt;
    % G(4:6,4:6) =  - Rbn;
    % G(7:9,1:3) = -skewMat(pn)*Rbn * dt;
    % G(7:9,4:6) =  - Rbn;
    % G(10:12,7:9) = eye(3)*dt;
    % G(13:15,10:12) = eye(3)*dt;
    G(1:3,1:3) =  - Rbn * dt;
    G(4:6,1:3) = -skewMat(vn)*Rbn * dt;
    G(4:6,4:6) =  - Rbn* dt;
    G(7:9,1:3) = -skewMat(pn)*Rbn * dt;
    G(7:9,4:6) =  - Rbn* dt;
    G(10:12,7:9) = eye(3) ;
    G(13:15,10:12) = eye(3) ;
    
    %G = G*double(dt);
end

== matlab function VB_RIFKF_GNSS_INS25/ISUS_RIEKF3/Error State Kalman Filter M2/Cal Q1/MATLAB Function1 ==
  data: Q output; dt input
function Q = fcn(dt)
    % G.block(0, 0, 3, 3) = -exp_so3(-w_hat * dt) * Jr_so3(-w_hat * dt) * dt;
    %    G.block(6, 3, 3, 3) = -R_Gtoi.transpose() * dt;
    %    G.block(3, 3, 3, 3) = -0.5 * R_Gtoi.transpose() * dt * dt;
    %    G.block(9, 6, 3, 3).setIdentity();
    %    G.block(12, 9, 3, 3).setIdentity();
    

    cov_dim = 12;
    Q = zeros(cov_dim,cov_dim);
%     noises_sigma_a_2 = 2.0000e-4^2;
%     noises_sigma_w_2 = 1.6968e-4^2;
%     noises_sigma_ab_2 = 3.0000e-4^2;
%     noises_sigma_wb_2 = 1.9393e-5^2;
    noises_sigma_a_2 = 0.001^2*1;
    %noises_sigma_w_2 = 0.0001^2;
    noises_sigma_w_2 = 0.0001^2;
    noises_sigma_ab_2 = 1.0000e-4^2*1;
    noises_sigma_wb_2 = 0.0002^2;
    % noises_sigma_mb_2 = 0.001^2;
    % noises_sigma_dtheta_2 = (1/57.3)^2;
    % noises_sigma_dwind_2 = 0.01^2;
    Q = diag([noises_sigma_w_2 / dt * ones(3,1); ...
                noises_sigma_a_2 / dt * ones(3,1); ...
                noises_sigma_wb_2 * dt * ones(3,1); ...
                noises_sigma_ab_2 * dt * ones(3,1); ...
                ]);
    

end

== matlab function VB_RIFKF_GNSS_INS25/ISUS_RIEKF3/Error State Kalman Filter M2/Extended Kalman Filter M1/Correct M1/Correct ==
  settings: updateMethod=DISCRETE  sampleTime=SampleTime
  data: x input; xNew output; P input; P output; yMeas input; R input; uMeas input; blockOrdering input; pM parameter; blockOrdering output
function [xNew,P,blockOrdering] = fcn(x,P,yMeas,R,uMeas,blockOrdering,pM)
% ekfCorrect Correction step for EKF
%
%   Copyright 2016-2021 The MathWorks, Inc.

%#codegen

% If measurement noise is time-varying then compute square-root
% factorization.
if pM.HasTimeVaryingR
   R = matlabshared.tracking.internal.svdPSD(R);
end

% Construct the function handle for measurement fcn
if pM.IsSimulinkFcn
    MeasurementFcnH_SL = str2func(pM.FcnName);
    if pM.HasAdditiveNoise
        MeasurementFcnH = @(fState)MeasurementFcnH_SL(fState);
    else
        MeasurementFcnH = @(fState,fMeasNoise)MeasurementFcnH_SL(fState,fMeasNoise);
    end
else
    MeasurementFcnH = str2func(pM.FcnName);
end

% Construct the function handle for measurement Jacobian fcn
if pM.HasJacobian
    if pM.IsSimulinkFcn
        MeasurementJacobianFcnH_SL = str2func(pM.JacobianFcnName);
        if pM.HasAdditiveNoise
            MeasurementJacobianFcnH = @(fState)MeasurementJacobianFcnH_SL(fState);
        else
            MeasurementJacobianFcnH = @(fState,fMeasNoise)MeasurementJacobianFcnH_SL(fState,fMeasNoise);
        end
    else
        MeasurementJacobianFcnH = str2func(pM.JacobianFcnName);
    end
else
    MeasurementJacobianFcnH = [];
end

% Handle (optional) extra input arguments of the measurement & jacobian fcns
switch pM.NumberOfExtraArgumentInports
    case 0
        extraArgs = {};
    case 1
        extraArgs = {uMeas};
    otherwise
        assert(false);
end

% Construct the corrector, perform the update
if pM.HasAdditiveNoise
    ekfCorrector = matlabshared.tracking.internal.EKFCorrectorAdditive();
else
    ekfCorrector = matlabshared.tracking.internal.EKFCorrectorNonAdditive();
end

% Check if dimensions and type of Measurement and Jacobian are correct
if pM.HasAdditiveNoise
   % Additive noise
   
   % MeasurementFcn
   ztry = MeasurementFcnH(x, extraArgs{:});
   
   if pM.IsSimulinkFcn
      hasError = (numel(ztry) ~= numel(yMeas));
   else
      hasError = (numel(ztry) ~= numel(yMeas)) || ~isa(ztry, class(x));
   end
   
   coder.internal.errorIf(...
      hasError,...
      'shared_tracking:ExtendedKalmanFilter:MeasurementNonMatchingSizeOrClass',...
      'MeasurementFcn');
   
   if pM.HasJacobian
      % MeasurementJacobianFcn
      Htry = MeasurementJacobianFcnH(x, extraArgs{:});
      isSizeNotCorrect = numel(yMeas) ~= size(Htry,1) || numel(x) ~= size(Htry,2);
      
      if pM.IsSimulinkFcn
         hasError = isSizeNotCorrect;
      else
         hasError = isSizeNotCorrect || ~isa(Htry, class(x));
      end
      
      coder.internal.errorIf(...
         hasError,...
         'shared_tracking:ExtendedKalmanFilter:MeasurementJacobianNonMatchingSizeOrClass',...
         'MeasurementJacobianFcn',numel(yMeas),numel(x));
   end   
else
   % Non-additive noise
   
   % MeasurementFcn
   ztry = MeasurementFcnH(...
      x, zeros(size(R,1),1,'like',x), ...
      extraArgs{:});   

   if pM.IsSimulinkFcn
      hasError = (numel(ztry) ~= numel(yMeas));
   else
      hasError = (numel(ztry) ~= numel(yMeas)) || ~isa(ztry, class(x));
   end
   
   coder.internal.errorIf(...
      hasError,...
      'shared_tracking:ExtendedKalmanFilter:MeasurementNonMatchingSizeOrClass',...
      'MeasurementFcn');
   
   if pM.HasJacobian
      % MeasurementJacobianFcn
      Htry = MeasurementJacobianFcnH(...
         x, zeros(size(R,1),1,'like',x), ...
         extraArgs{:});
      
      isSizeNotCorrect = numel(yMeas) ~= size(Htry,1) || numel(x) ~= size(Htry,2);     
      
      if pM.IsSimulinkFcn
         hasError = isSizeNotCorrect;
      else
         hasError = isSizeNotCorrect || ~isa(Htry, class(x));
      end
      
      coder.internal.errorIf(...
         hasError,...
         'shared_tracking:ExtendedKalmanFilter:MeasurementJacobianNonMatchingSizeOrClass',...
         'MeasurementJacobianFcn',numel(yMeas),numel(x));
   end
end
% Measurement wrapping
ekfCorrector.HasMeasurementWrapping = pM.HasWrapping;

xNew = zeros(size(x),'like',x); %#ok<PREALL>
% wk = 0;
[xNew,P] = ekfCorrector.correct(...
        yMeas,R,x,P,MeasurementFcnH,MeasurementJacobianFcnH,extraArgs{:});
end

== matlab function VB_RIFKF_GNSS_INS25/ISUS_RIEKF3/Error State Kalman Filter M2/Extended Kalman Filter M1/Correct M1/MATLAB Function ==
  data: u input; y output
function y = fcn(u)

y = tril(u);

== matlab function VB_RIFKF_GNSS_INS25/ISUS_RIEKF3/Error State Kalman Filter M2/Extended Kalman Filter M1/Correct M1/Subsystem2/MATLAB Function1 ==
  data: u input; y output; X input; ISUS_flag input
function y = fcn(u, X, ISUS_flag)
if ISUS_flag == 0
    y = X;
else
     y = u;
    %y(1:9,1:9) = u;
end

== matlab function VB_RIFKF_GNSS_INS25/ISUS_RIEKF3/Error State Kalman Filter M2/Extended Kalman Filter M1/Correct M1/innovation calculation/MATLAB Function ==
  data: u input; y output
function y = fcn(u)

y = u*u';

== matlab function VB_RIFKF_GNSS_INS25/No.1_Sensor_Data_Process/IMU_Data_Process/accl_preprocessing2/MATLAB Function3 ==
  data: curr_input input; curr_output output single; sample_freq input; cutoff_freq input
function curr_output = second_LPF_Butter_x(curr_input,sample_freq,cutoff_freq)
   persistent input_x;
   persistent output_x;

   if isempty(input_x)
       input_x = [0;0;0];
   end
   
   if isempty(output_x)
       output_x = [0;0;0];
   end
    B = [0,0,0];
    A = [0,0,0];
    M_PI_F = 3.1415926;
	fr = sample_freq / cutoff_freq;
	ohm = tan( M_PI_F / fr );
	c = 1.0 + 2.0 * cos( M_PI_F / 4.0 ) * ohm + ohm * ohm;
	B(1) = ohm * ohm / c;
	B(2) = 2.0 * B(1);
	B(3) = B(1);
	A(1) = 2.0 * ( ohm * ohm - 1.0) / c;
	A(2) = (1.0 - 2.0 * cos( M_PI_F / 4.0 ) * ohm + ohm * ohm) / c;
	%/*获取最新输入*/
	input_x(3) = curr_input;
	%/* Butterworth */
	output_x(3) =B(1) * input_x(3) + B(2) * input_x(2) +B(3) * input_x(1) - A(1) * output_x(2) - A(2) * output_x(1);
	curr_output = single(output_x(3));
   % /* 输入序列保存 */
	input_x(1) = input_x(2);
	input_x(2) = input_x(3);
	%/*输出序列保存 */
	output_x(1) = output_x(2);
	output_x(2) = output_x(3);

== matlab function VB_RIFKF_GNSS_INS25/ISUS_RIEKF3/Error State Kalman Filter M2/Extended Kalman Filter M1/Output/MATLAB Function ==
  data: S input; P output
function P = fcn(S)
    
    % Get back Covariance from Square-root Covariance
    P = S*S';
    %P = 1/2*(S+S');
    
end

== matlab function VB_RIFKF_GNSS_INS25/ISUS_RIEKF3/Error State Kalman Filter M2/Extended Kalman Filter M1/Predict/Predict ==
  settings: updateMethod=DISCRETE  sampleTime=SampleTime
  data: x input; xNew output; P input; Q input; uState input; unused input; P output; pS parameter
function [xNew,P] = fcn(x,P,Q,uState,~,pS)
% ekfCorrect Prediction step for EKF
%
%   Copyright 2016-2021 The MathWorks, Inc.

%#codegen

% If process noise is time-varying then compute square-root
% factorization.
if pS.HasTimeVaryingQ
   Q = matlabshared.tracking.internal.svdPSD(Q);
end

% Construct fcn handles
if pS.IsSimulinkFcn
    StateTransitionJacobianFcnH_SL = str2func(pS.FcnName);
    if pS.HasAdditiveNoise
        StateTransitionFcnH = @(fState)StateTransitionJacobianFcnH_SL(fState);
    else
        StateTransitionFcnH = @(fState,fProcNoise)StateTransitionJacobianFcnH_SL(fState,fProcNoise);
    end
else
    StateTransitionFcnH = str2func(pS.FcnName);
end
if pS.HasJacobian
    if pS.IsSimulinkFcn
        StateTransitionJacobianFcnH_SL = str2func(pS.JacobianFcnName);
        if pS.HasAdditiveNoise
            StateTransitionJacobianFcnH = @(fState)StateTransitionJacobianFcnH_SL(fState);
        else
            StateTransitionJacobianFcnH = @(fState,fProcNoise)StateTransitionJacobianFcnH_SL(fState,fProcNoise);
        end
    else
        StateTransitionJacobianFcnH = str2func(pS.JacobianFcnName);
    end
else
    StateTransitionJacobianFcnH = [];
end

switch pS.NumberOfExtraArgumentInports
    case 0
        extraArgs = {};
    case 1
        extraArgs = {uState};
    otherwise
        assert(false);
end

% Check if dimensions and type of State and Jacobian are correct
if pS.HasAdditiveNoise
   % Additive noise
   
   % StateTransitionFcn
   xTry = StateTransitionFcnH(x, extraArgs{:});
   
   if pS.IsSimulinkFcn
      hasError = any(size(x) ~= size(xTry));
   else
      hasError = any(size(x) ~= size(xTry)) || ~isa(xTry, class(x));
   end
   
   coder.internal.errorIf(...
      hasError,...
      'shared_tracking:ExtendedKalmanFilter:StateNonMatchingSizeOrClass',...
      'StateTransitionFcn', 'State', numel(x));
   
   if pS.HasJacobian
      % Jacobian
      F = StateTransitionJacobianFcnH(x, extraArgs{:});
      % F needs to be square
      isSizeNotCorrect = ~all(size(F) == numel(x));
      
      if pS.IsSimulinkFcn
         hasError = isSizeNotCorrect;
      else
         hasError = isSizeNotCorrect || ~isa(F, class(x));
      end
      
      coder.internal.errorIf(...
         hasError,...
         'shared_tracking:ExtendedKalmanFilter:StateTransitionJacobianNonMatchingSizeOrClass',...
         'StateTransitionJacobianFcn', numel(x));
   end
else
   % Non-additive noise
   
   % StateTransitionFcn
   xTry = StateTransitionFcnH(x, zeros(size(Q,1),1,'like',x),extraArgs{:});
   
   if pS.IsSimulinkFcn
      hasError = any(size(x) ~= size(xTry));
   else
      hasError = any(size(x) ~= size(xTry)) || ~isa(xTry, class(x));
   end
   
   coder.internal.errorIf(...
      hasError,...
      'shared_tracking:ExtendedKalmanFilter:StateNonMatchingSizeOrClass',...
      'StateTransitionFcn', 'State', numel(x))
   
   if pS.HasJacobian
      % Jacobian
      F = StateTransitionJacobianFcnH(x, zeros(size(Q,1),1,'like',x),extraArgs{:});
      % F needs to be square
      isSizeNotCorrect = ~all(size(F) == numel(x));
      
      if pS.IsSimulinkFcn
         hasError = isSizeNotCorrect;
      else
         hasError = isSizeNotCorrect || ~isa(F, class(x));
      end
       
      coder.internal.errorIf(...
         hasError,...
         'shared_tracking:ExtendedKalmanFilter:StateTransitionJacobianNonMatchingSizeOrClass',...
         'StateTransitionJacobianFcn', numel(x));
   end
end

xNew = zeros(size(x),'like',x); %#ok<PREALL>

if pS.HasAdditiveNoise
    [xNew,P] = matlabshared.tracking.internal.EKFPredictorAdditive.predict(...
        Q,x,P,StateTransitionFcnH,StateTransitionJacobianFcnH,extraArgs{:});
else    
    [xNew,P] = matlabshared.tracking.internal.EKFPredictorNonAdditive.predict(...
        Q,x,P,StateTransitionFcnH,StateTransitionJacobianFcnH,extraArgs{:});
end
end

== matlab function VB_RIFKF_GNSS_INS25/ISUS_RIEKF3/Error State Kalman Filter M2/MATLAB Function ==
  data: u input; dp output size=3; dv output size=3; dtheta output size=3; da output size=3; dg output size=3
function [dp,dv,dtheta,da,dg] = fcn(u)
    dtheta = u(1:3);
    dv = u(4:6);
    dp = u(7:9);
    dg = u(10:12);
    da = u(13:15);

end
